simulink model "emo_1wr8_exec"  (Simulink 3.00)
libraries: execlib x6

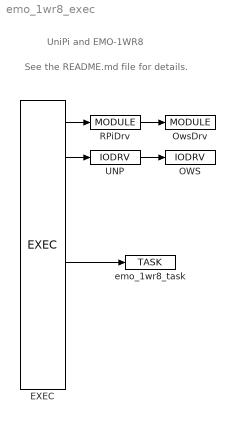
== system emo_1wr8_exec ==
  note: UniPi and EMO-1WR8
  note: See the README.md file for details.
  EXEC : execlib/EXEC  target=Generic target device  tick=0.01  ntick0=1  ntick1=50  ntick2=100  ntick3=1200  pri0=5  pri1=9  pri2=13  pri3=18
  OWS : execlib/IODRV  module=OwsDrv  classname=OwsDrv  cfgname=emo_1wr8_owscfg.rio  factor=5  stack=10240  pri=3  timer=off
  OwsDrv : execlib/MODULE
  RPiDrv : execlib/MODULE
  UNP : execlib/IODRV  module=RPiDrv  classname=UnpDrv  factor=1  stack=10240  pri=3  timer=off
  emo_1wr8_task : execlib/TASK  factor=1  start=0  stop=1  stack=10240  MDLOPEN=on
  wires:
  EXEC/1 -> RPiDrv/1
  EXEC/2 -> UNP/1
  EXEC/5 -> emo_1wr8_task/1
  RPiDrv/1 -> OwsDrv/1
  UNP/1 -> OWS/1
